simulink model "Accelerator_Pedal_Position_Sensor"  (R2022b)
settings: Solver=FixedStepAuto  StartTime=0.0  StopTime=10.0  RelTol=1e-3
settings Model: Creator=yasso  LastModifiedBy=yasso
settings DataIOCC: ExternalInput=[t, AcceleratorPedalPosition1,AcceleratorPedalPosition2]  LoadExternalInput=on

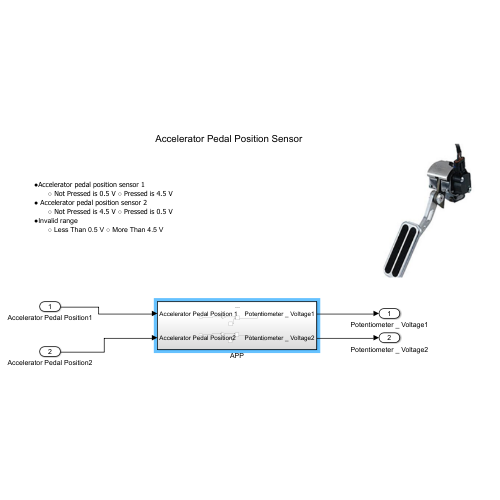
[thumbnail: Simulink's stored preview of the top-level diagram]
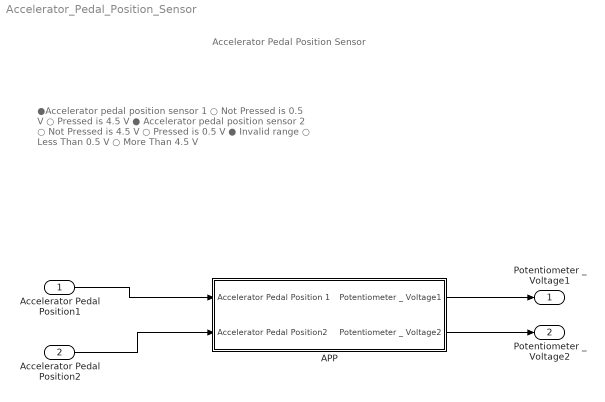
== system Accelerator_Pedal_Position_Sensor ==
  note: ●Accelerator pedal position sensor 1
      | ○ Not Pressed is 0.5 V ○ Pressed is 4.5 V
      | ● Accelerator pedal position sensor 2
      | ○ Not Pressed is 4.5 V ○ Pressed is 0.5 V
      | ● Invalid range
      | ○ Less Than 0.5 V ○ More Than 4.5 V
  note: Accelerator Pedal Position Sensor
  Accelerator Pedal Position1 : Inport
  Accelerator Pedal Position2 : Inport  Port=2
  APP : Subsystem
  Potentiometer _ Voltage1 : Outport
  Potentiometer _ Voltage2 : Outport  Port=2
  wires:
  Accelerator Pedal Position1/1 -> APP/1(Accelerator Pedal Position 1)
  Accelerator Pedal Position2/1 -> APP/2(Accelerator Pedal Position2)
  APP/1(Potentiometer _ Voltage1) -> Potentiometer _ Voltage1/1
  APP/2(Potentiometer _ Voltage2) -> Potentiometer _ Voltage2/1

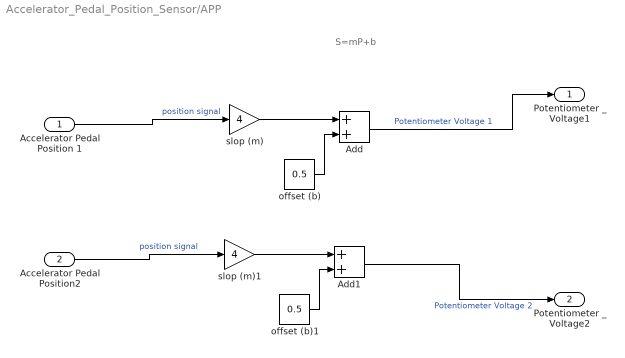
== system Accelerator_Pedal_Position_Sensor/APP ==
  note: S=mP+b
  Accelerator Pedal Position 1 : Inport
  Accelerator Pedal Position2 : Inport  Port=2
  Add : Sum
  Add1 : Sum
  offset (b) : Constant  Value=0.5
  offset (b)1 : Constant  Value=0.5
  slop (m) : Gain  Gain=4
  slop (m)1 : Gain  Gain=4
  Potentiometer _ Voltage1 : Outport
  Potentiometer _ Voltage2 : Outport  Port=2
  wires:
  Accelerator Pedal Position 1/1 -> slop (m)/1  "position signal"
  slop (m)/1 -> Add/1
  offset (b)/1 -> Add/2
  Add/1 -> Potentiometer _ Voltage1/1  "Potentiometer Voltage 1"
  Add1/1 -> Potentiometer _ Voltage2/1  "Potentiometer Voltage 2"
  offset (b)1/1 -> Add1/2
  slop (m)1/1 -> Add1/1
  Accelerator Pedal Position2/1 -> slop (m)1/1  "position signal"
